simulink model "Projekt_Kessel_gesteuert"  (Simulink 4.00)
settings: Solver=ode45  StartTime=0.0  StopTime=inf  RelTol=1e-3
libraries: simulink3 x6
settings Model: LastModifiedBy=Administrator  BlockReductionOpt=off

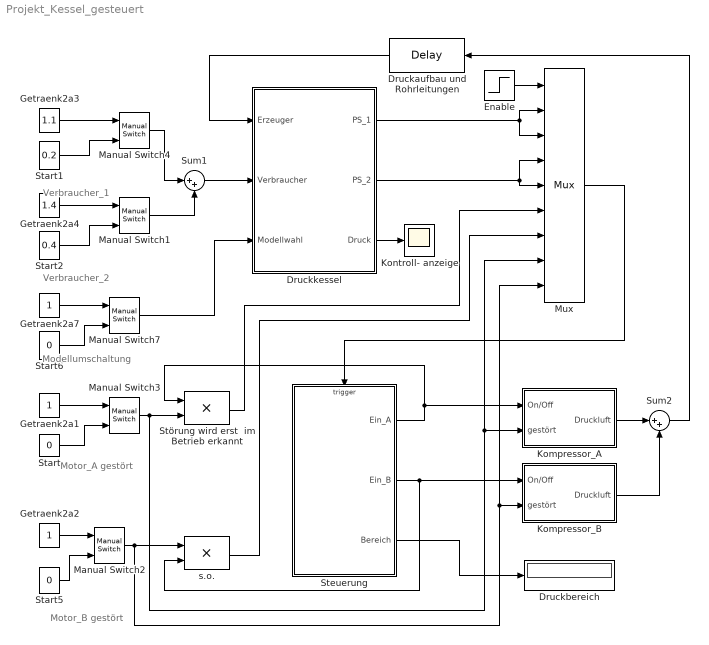
== system Projekt_Kessel_gesteuert ==
  note: Motor_A gestört
  note: Verbraucher_1
  note: Verbraucher_2
  note: Motor_B gestört
  note: Modellumschaltung
  Druckaufbau und Rohrleitungen : TransportDelay  Orientation=left  DelayTime=2  InitialInput=0  BufferSize=1024  PadeOrder=0
  Druckbereich : Display
      settings: Format=short
  Druckkessel : Subsystem
      settings: RTWFcnNameOpts=Auto  RTWFileNameOpts=Auto
  Enable : Step  Time=0.5  Before=0  After=1  SampleTime=0
  Getraenk2a1 : Constant  Value=1
  Getraenk2a2 : Constant  Value=1
  Getraenk2a3 : Constant  Value=1.1
  Getraenk2a4 : Constant  Value=1.4
  Getraenk2a7 : Constant  Value=1
  Kompressor_A : Subsystem
      settings: RTWFcnNameOpts=Auto  RTWFileNameOpts=Auto
  Kompressor_B : Subsystem
      settings: RTWFcnNameOpts=Auto  RTWFileNameOpts=Auto
  Kontroll- anzeige : Scope
      settings: TimeRange=10  YMin=2.84  YMax=3.04  SaveToWorkspace=off  SaveName=ScopeData  LimitDataPoints=on  MaxDataPoints=5000
  Manual Switch1 : simulink3/Nonlinear/Manual Switch  sw=0  action=0
  Manual Switch2 : simulink3/Nonlinear/Manual Switch  sw=0  action=0
  Manual Switch3 : simulink3/Nonlinear/Manual Switch  sw=0  action=0
  Manual Switch4 : simulink3/Nonlinear/Manual Switch  sw=1  action=0
  Manual Switch7 : simulink3/Nonlinear/Manual Switch  sw=1  action=0
  Mux : Mux  Inputs=9
      settings: DisplayOption=none
  Start : Constant  Value=0
  Start1 : Constant  Value=0.2
  Start2 : Constant  Value=0.4
  Start5 : Constant  Value=0
  Start6 : Constant  Value=0
  Steuerung : Stateflow chart  TreatAsAtomicUnit=on
      settings: RTWFcnNameOpts=Auto  RTWFileNameOpts=Auto
  Störung wird erst  im Betrieb erkannt : Product  Inputs=2  Multiplication=Element-wise(.*)  SaturateOnIntegerOverflow=on
  Sum1 : Sum  Inputs=|++  SaturateOnIntegerOverflow=on
  Sum2 : Sum  Inputs=|++  SaturateOnIntegerOverflow=on
  s.o. : Product  Inputs=2  Multiplication=Element-wise(.*)  SaturateOnIntegerOverflow=on
  wires:
  Enable/1 -> Mux/1
  Mux/1 -> Steuerung/Trigger
  Getraenk2a2/1 -> Manual Switch2/1
  Start/1 -> Manual Switch3/2
  Getraenk2a1/1 -> Manual Switch3/1
  Start1/1 -> Manual Switch4/2
  Getraenk2a3/1 -> Manual Switch4/1
  Start2/1 -> Manual Switch1/2
  Getraenk2a4/1 -> Manual Switch1/1
  Steuerung/3(Bereich) -> Druckbereich/1
  Steuerung/1(Ein_A) -> Störung wird erst  im Betrieb erkannt/1, Kompressor_A/1(On/Off)
  Steuerung/2(Ein_B) -> s.o./2, Kompressor_B/1(On/Off)
  Druckaufbau und Rohrleitungen/1 -> Druckkessel/1(Erzeuger)
  Sum2/1 -> Druckaufbau und Rohrleitungen/1
  Manual Switch3/1 -> Störung wird erst  im Betrieb erkannt/2, Mux/8, Kompressor_A/2(gestört)
  Störung wird erst  im Betrieb erkannt/1 -> Mux/6
  s.o./1 -> Mux/7
  Sum1/1 -> Druckkessel/2(Verbraucher)
  Druckkessel/3(Druck) -> Kontroll- anzeige/1
  Manual Switch1/1 -> Sum1/2
  Start6/1 -> Manual Switch7/2
  Getraenk2a7/1 -> Manual Switch7/1
  Druckkessel/2(PS_2) -> Mux/4, Mux/5
  Druckkessel/1(PS_1) -> Mux/2, Mux/3
  Kompressor_A/1(Druckluft) -> Sum2/1
  Kompressor_B/1(Druckluft) -> Sum2/2
  Manual Switch7/1 -> Druckkessel/3(Modellwahl)
  Start5/1 -> Manual Switch2/2
  Manual Switch2/1 -> s.o./1, Mux/9, Kompressor_B/2(gestört)
  Manual Switch4/1 -> Sum1/1

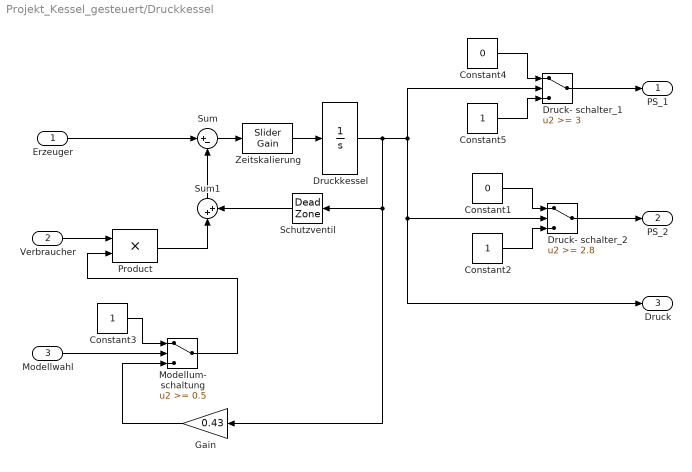
== system Projekt_Kessel_gesteuert/Druckkessel ==
  Erzeuger : Inport  Port=1
  Verbraucher : Inport  Port=2
  Modellwahl : Inport  Port=3
  Constant1 : Constant  Value=0
  Constant2 : Constant  Value=1
  Constant3 : Constant  Value=1
  Constant4 : Constant  Value=0
  Constant5 : Constant  Value=1
  Druck- schalter_1 : Switch  Threshold=3
  Druck- schalter_2 : Switch  Threshold=2.8
  Druckkessel : Integrator  ExternalReset=none  InitialConditionSource=internal  InitialCondition=3.5  LimitOutput=on  UpperSaturationLimit=10  LowerSaturationLimit=0  ShowSaturationPort=off  ShowStatePort=off  AbsoluteTolerance=auto
  Gain : Gain  Orientation=left  Gain=0.43  Multiplication=Element-wise(K.*u)  SaturateOnIntegerOverflow=on
  Modellum- schaltung : Switch  Threshold=0.5
  Product : Product  Inputs=2  Multiplication=Element-wise(.*)  SaturateOnIntegerOverflow=on
  Schutzventil : DeadZone  Orientation=left  LowerValue=-1.  UpperValue=5  SaturateOnIntegerOverflow=on  LinearizeAsGain=on
  Sum : Sum  Inputs=|+-  SaturateOnIntegerOverflow=on
  Sum1 : Sum  Orientation=up  Inputs=|++  SaturateOnIntegerOverflow=on
  Zeitskalierung : simulink3/Math/Slider Gain  low=0  gain=0.01  high=0.2
  PS_1 : Outport  Port=1
  PS_2 : Outport  Port=2
  Druck : Outport  Port=3
  wires:
  Druckkessel/1 -> Druck- schalter_1/2, Druck- schalter_2/2, Druck/1, Schutzventil/1, Gain/1
  Constant4/1 -> Druck- schalter_1/1
  Constant5/1 -> Druck- schalter_1/3
  Druck- schalter_1/1 -> PS_1/1
  Constant1/1 -> Druck- schalter_2/1
  Constant2/1 -> Druck- schalter_2/3
  Druck- schalter_2/1 -> PS_2/1
  Sum/1 -> Zeitskalierung/1
  Zeitskalierung/1 -> Druckkessel/1
  Verbraucher/1 -> Product/1
  Schutzventil/1 -> Sum1/2
  Sum1/1 -> Sum/2
  Product/1 -> Sum1/1
  Modellwahl/1 -> Modellum- schaltung/2
  Constant3/1 -> Modellum- schaltung/1
  Modellum- schaltung/1 -> Product/2
  Erzeuger/1 -> Sum/1
  Gain/1 -> Modellum- schaltung/3

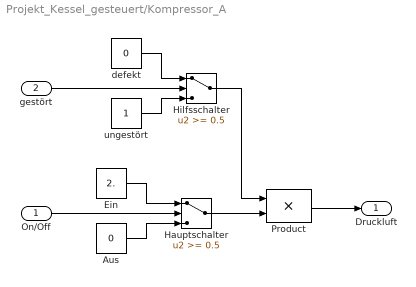
== system Projekt_Kessel_gesteuert/Kompressor_A ==
  On/Off : Inport  Port=1
  gestört : Inport  Port=2
  Aus : Constant  Value=0
  Ein : Constant  Value=2.
  Hauptschalter : Switch  Threshold=0.5
  Hilfsschalter : Switch  Threshold=0.5
  Product : Product  Inputs=2  Multiplication=Element-wise(.*)  SaturateOnIntegerOverflow=on
  defekt : Constant  Value=0
  ungestört : Constant  Value=1
  Druckluft : Outport  Port=1
  wires:
  Ein/1 -> Hauptschalter/1
  Aus/1 -> Hauptschalter/3
  On/Off/1 -> Hauptschalter/2
  defekt/1 -> Hilfsschalter/1
  ungestört/1 -> Hilfsschalter/3
  gestört/1 -> Hilfsschalter/2
  Hauptschalter/1 -> Product/2
  Product/1 -> Druckluft/1
  Hilfsschalter/1 -> Product/1

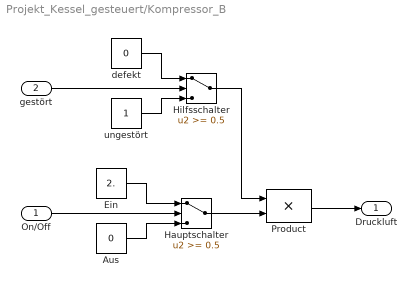
== system Projekt_Kessel_gesteuert/Kompressor_B ==
  On/Off : Inport  Port=1
  gestört : Inport  Port=2
  Aus : Constant  Value=0
  Ein : Constant  Value=2.
  Hauptschalter : Switch  Threshold=0.5
  Hilfsschalter : Switch  Threshold=0.5
  Product : Product  Inputs=2  Multiplication=Element-wise(.*)  SaturateOnIntegerOverflow=on
  defekt : Constant  Value=0
  ungestört : Constant  Value=1
  Druckluft : Outport  Port=1
  wires:
  Ein/1 -> Hauptschalter/1
  Aus/1 -> Hauptschalter/3
  On/Off/1 -> Hauptschalter/2
  defekt/1 -> Hilfsschalter/1
  ungestört/1 -> Hilfsschalter/3
  gestört/1 -> Hilfsschalter/2
  Hauptschalter/1 -> Product/2
  Product/1 -> Druckluft/1
  Hilfsschalter/1 -> Product/1

== stateflow chart Steuerung ==
  state Kessel [parallel]
    state Druck_hoch
      entry:Bereich=3;
    state Druck_mittel
      en:Bereich=2;
    state Druck_tief
      en:Bereich=1;
    Druck_hoch -> Druck_mittel : PS_1_s/einschalten();
    Druck_mittel -> Druck_tief : PS_2_s/Ein;
    Druck_tief -> Druck_mittel : PS_2_f/abschalten();
    Druck_mittel -> Druck_hoch : PS_1_f/Aus;
    (default) -> Druck_hoch
  state Motor_A [parallel]
    state Off
      en:Ein_A=0;
    state On
      en:Ein_A=1;
    state Down
      en:Err_A=1;
      exit:Err_A=0;
    Motor_A.Off -> Motor_A.On : Ein
    Motor_A.Down -> (junction 20) : OK_A
    (default) -> Motor_A.Off
    Motor_A.On -> Motor_A.Off : Aus/Flag=1;
    Motor_A.On -> Motor_A.Down : Down_A/Ein;
    (junction 20) -> Motor_A.Off
    (junction 20) -> Motor_A.On : [(Bereich==1) | (Bereich==2 & Err_B==1)]
  state Motor_B [parallel]
    state Off
      en:Ein_B=0;
    state Down
      en:Err_B=1;
      exit:Err_B=0;
    state On
      en:Ein_B=1;
    Motor_B.On -> Motor_B.Off : Aus/Flag=0;
    Motor_B.On -> Motor_B.Down : Down_B/Ein;
    Motor_B.Down -> (junction 21) : OK_B
    (default) -> Motor_B.Off
    Motor_B.Off -> Motor_B.On : Ein
    (junction 21) -> Motor_B.On : [(Bereich==1) | (Bereich==2 & Err_A==1)]
    (junction 21) -> Motor_B.Off
  state einschalten() [function]
    (junction 17) -> (junction 18) : [Flag==0]{send(Ein,Motor_A);}
    (junction 17) -> (junction 19) : [Flag==1]{send(Ein,Motor_B);}
    (default) -> (junction 22)
    (junction 22) -> (junction 17)
    (junction 22) -> (junction 23) : [Err_A+Err_B>=1]{send(Ein);}
  state abschalten() [function]
    (junction 25) -> (junction 24) : [Err_A==1]
    (junction 25) -> (junction 26)
    (default) -> (junction 25)
    (junction 25) -> (junction 27) : [Err_B==1]
    (junction 26) -> (junction 28) : [Flag==1]{send(Aus,Motor_B);}
    (junction 26) -> (junction 29) : [Flag==0]{send(Aus,Motor_A);}
  (default) -> Kessel
  (default) -> Motor_A
  (default) -> Motor_B
  data: Ein_A output int16; Ein_B output int16; Bereich output int16 =3; Flag local int16; Err_A local int16; Err_B local int16
  events: Enable input RISING_EDGE_EVENT; PS_1_s input RISING_EDGE_EVENT; PS_1_f input FALLING_EDGE_EVENT; PS_2_s input RISING_EDGE_EVENT; PS_2_f input FALLING_EDGE_EVENT; Ein local EITHER_EDGE_EVENT; Aus local EITHER_EDGE_EVENT; Down_A input RISING_EDGE_EVENT; Down_B input RISING_EDGE_EVENT; OK_A input FALLING_EDGE_EVENT; OK_B input EITHER_EDGE_EVENT
